simulink model "final"  (R2023a)
settings: Solver=FixedStepAuto  StartTime=0.0  StopTime=25  FixedStep=0.001  RelTol=1e-3
settings Model: Creator=asus  LastModifiedBy=asus

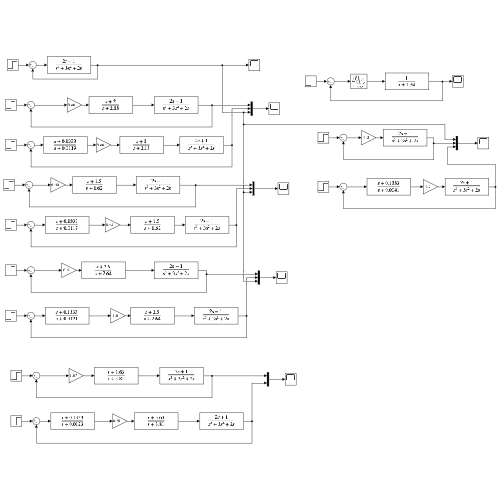
[thumbnail: Simulink's stored preview of the top-level diagram]
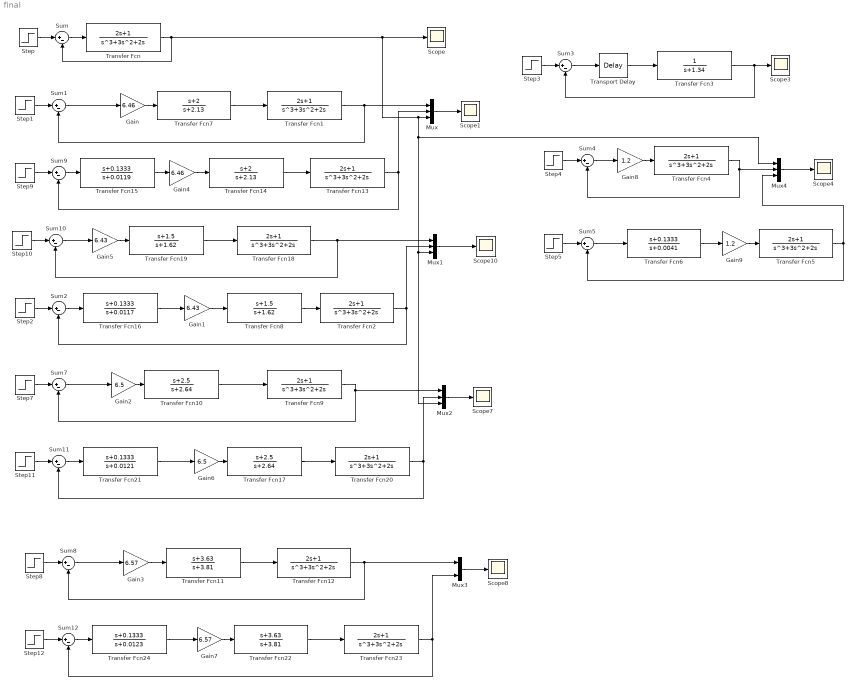
== system final ==
  Gain : Gain  Gain=6.46
  Gain1 : Gain  Gain=6.43
  Gain2 : Gain  Gain=6.5
  Gain3 : Gain  Gain=6.57
  Gain4 : Gain  Gain=6.46
  Gain5 : Gain  Gain=6.43
  Gain6 : Gain  Gain=6.5
  Gain7 : Gain  Gain=6.57
  Gain8 : Gain  Gain=1.2
  Gain9 : Gain  Gain=1.2
  Mux{,1..2,4} (4 alike) : Mux  Inputs=3
  Mux3 : Mux  Inputs=2
  Scope{,1,3..4,7..8,10} (7 alike) : Scope
  Step{,1..5,7..12} (12 alike) : Step  Time=0  SampleTime=0
  Sum{,1..5,7..12} (12 alike) : Sum  Inputs=|+-
  Transfer Fcn{,1..2,4..5,9,12..13,18,20,23} (11 alike) : TransferFcn  Numerator=[2 1]  Denominator=[1 3 2 0]
  Transfer Fcn10 : TransferFcn  Numerator=[1 2.5]  Denominator=[1 2.64]
  Transfer Fcn11 : TransferFcn  Numerator=[1 3.63]  Denominator=[1 3.81]
  Transfer Fcn14 : TransferFcn  Numerator=[1 2]  Denominator=[1 2.13]
  Transfer Fcn15 : TransferFcn  Numerator=[1 0.1333]  Denominator=[1 0.0119]
  Transfer Fcn16 : TransferFcn  Numerator=[1 0.1333]  Denominator=[1 0.0117]
  Transfer Fcn17 : TransferFcn  Numerator=[1 2.5]  Denominator=[1 2.64]
  Transfer Fcn19 : TransferFcn  Numerator=[1 1.5]  Denominator=[1 1.62]
  Transfer Fcn21 : TransferFcn  Numerator=[1 0.1333]  Denominator=[1 0.0121]
  Transfer Fcn22 : TransferFcn  Numerator=[1 3.63]  Denominator=[1 3.81]
  Transfer Fcn24 : TransferFcn  Numerator=[1 0.1333]  Denominator=[1 0.0123]
  Transfer Fcn3 : TransferFcn  Denominator=[1 1.34]
  Transfer Fcn6 : TransferFcn  Numerator=[1 0.1333]  Denominator=[1 0.0041]
  Transfer Fcn7 : TransferFcn  Numerator=[1 2]  Denominator=[1 2.13]
  Transfer Fcn8 : TransferFcn  Numerator=[1 1.5]  Denominator=[1 1.62]
  Transport Delay : TransportDelay  DelayTime=0.2
  wires:
  Transfer Fcn/1 -> Sum/2, Mux4/1, Mux2/3, Mux1/3, Mux/3, Scope/1
  Sum/1 -> Transfer Fcn/1
  Step/1 -> Sum/1
  Step1/1 -> Sum1/1
  Transfer Fcn1/1 -> Mux/1, Sum1/2
  Transfer Fcn7/1 -> Transfer Fcn1/1
  Sum1/1 -> Gain/1
  Gain/1 -> Transfer Fcn7/1
  Transfer Fcn8/1 -> Transfer Fcn2/1
  Transfer Fcn2/1 -> Mux1/2, Sum2/2
  Gain1/1 -> Transfer Fcn8/1
  Step2/1 -> Sum2/1
  Transfer Fcn10/1 -> Transfer Fcn9/1
  Step7/1 -> Sum7/1
  Sum7/1 -> Gain2/1
  Gain2/1 -> Transfer Fcn10/1
  Transfer Fcn9/1 -> Mux2/1, Sum7/2
  Transfer Fcn11/1 -> Transfer Fcn12/1
  Gain3/1 -> Transfer Fcn11/1
  Sum8/1 -> Gain3/1
  Step8/1 -> Sum8/1
  Transfer Fcn12/1 -> Mux3/1, Sum8/2
  Transfer Fcn14/1 -> Transfer Fcn13/1
  Transfer Fcn13/1 -> Mux/2, Sum9/2
  Gain4/1 -> Transfer Fcn14/1
  Step9/1 -> Sum9/1
  Sum9/1 -> Transfer Fcn15/1
  Transfer Fcn15/1 -> Gain4/1
  Sum2/1 -> Transfer Fcn16/1
  Transfer Fcn16/1 -> Gain1/1
  Transfer Fcn19/1 -> Transfer Fcn18/1
  Step10/1 -> Sum10/1
  Gain5/1 -> Transfer Fcn19/1
  Transfer Fcn18/1 -> Mux1/1, Sum10/2
  Sum10/1 -> Gain5/1
  Transfer Fcn17/1 -> Transfer Fcn20/1
  Gain6/1 -> Transfer Fcn17/1
  Step11/1 -> Sum11/1
  Transfer Fcn20/1 -> Mux2/2, Sum11/2
  Sum11/1 -> Transfer Fcn21/1
  Transfer Fcn21/1 -> Gain6/1
  Gain7/1 -> Transfer Fcn22/1
  Transfer Fcn23/1 -> Mux3/2, Sum12/2
  Sum12/1 -> Transfer Fcn24/1
  Transfer Fcn22/1 -> Transfer Fcn23/1
  Step12/1 -> Sum12/1
  Transfer Fcn24/1 -> Gain7/1
  Step3/1 -> Sum3/1
  Sum3/1 -> Transport Delay/1
  Transfer Fcn3/1 -> Sum3/2, Scope3/1
  Transport Delay/1 -> Transfer Fcn3/1
  Transfer Fcn4/1 -> Mux4/2, Sum4/2
  Sum4/1 -> Gain8/1
  Step4/1 -> Sum4/1
  Gain8/1 -> Transfer Fcn4/1
  Step5/1 -> Sum5/1
  Gain9/1 -> Transfer Fcn5/1
  Transfer Fcn5/1 -> Mux4/3, Sum5/2
  Sum5/1 -> Transfer Fcn6/1
  Transfer Fcn6/1 -> Gain9/1
  Mux/1 -> Scope1/1
  Mux1/1 -> Scope10/1
  Mux2/1 -> Scope7/1
  Mux3/1 -> Scope8/1
  Mux4/1 -> Scope4/1
